simulink model "fixed_point_filter_CustArch_v9"  (R2020a)
settings: Solver=FixedStepAuto  StartTime=0  StopTime=60.5525  RelTol=1e-3
model workspace (MAT data in the model file):
  a = 0
undefined symbols (not defined in the file): fs
libraries: dsparch4 x2
settings Model: MinMaxOverflowLogging=MinMaxAndOverflow  FPTRunName=EmbeddedRun  FPTShortcutValueString='{{},{''BaselineRun_3'',1,1,1,''BaselineRun_3'','''',{},''M'',''D'',''''},{''EmbeddedRun'',1,1,1,''EmbeddedRun'','''',{},''M'','''',''''},{''BaselineRun'',1,1,1,''BaselineRun'','''',{},''M'',''D'',''''},{''BaselineRun_2'',1,1,1,''BaselineRun_2'','''',{},''M'',''D'',''''},{''EmbeddedRun_2'',1,1,1,''EmbeddedRun_2'','''',{},''M'','''',''''},{''BaselineRun_4'',1,1,1,''BaselineRun_4'','''',{},''M'',''D'',''''},{''BaselineRun_7'',1,1,1,''BaselineRun_7'','''',{},''M'',''D'',''''}}'  SimulationMode=rapid-accelerator  Creator=sbuccelli  LastModifiedBy=diflo
settings DataIOCC: SaveOutput=off  SaveTime=off
settings OptimizationCC: BlockReduction=off  ConditionallyExecuteInputs=off  DefaultParameterBehavior=Inlined
settings DebuggingCC: SignalRangeChecking=error  AlgebraicLoopMsg=error  SingleTaskRateTransMsg=error  IntegerOverflowMsg=none  ParameterDowncastMsg=none  ParameterOverflowMsg=none  ParameterPrecisionLossMsg=none  IntegerSaturationMsg=none
settings HardwareCC: ProdBitPerPointer=32  ProdBitPerSizeT=32  ProdBitPerPtrDiffT=32  ProdLargestAtomicFloat=None  ProdIntDivRoundTo=Undefined  ProdEndianess=Unspecified  ProdWordSize=32  ProdHWDeviceType=ASIC/FPGA->ASIC/FPGA  TargetBitPerPointer=64  TargetBitPerSizeT=64  TargetBitPerPtrDiffT=64  TargetLongLongMode=on  TargetIntDivRoundTo=Zero  TargetEndianess=LittleEndian  TargetWordSize=64  TargetHWDeviceType=Custom Processor->MATLAB Host Computer  ProdEqTarget=off

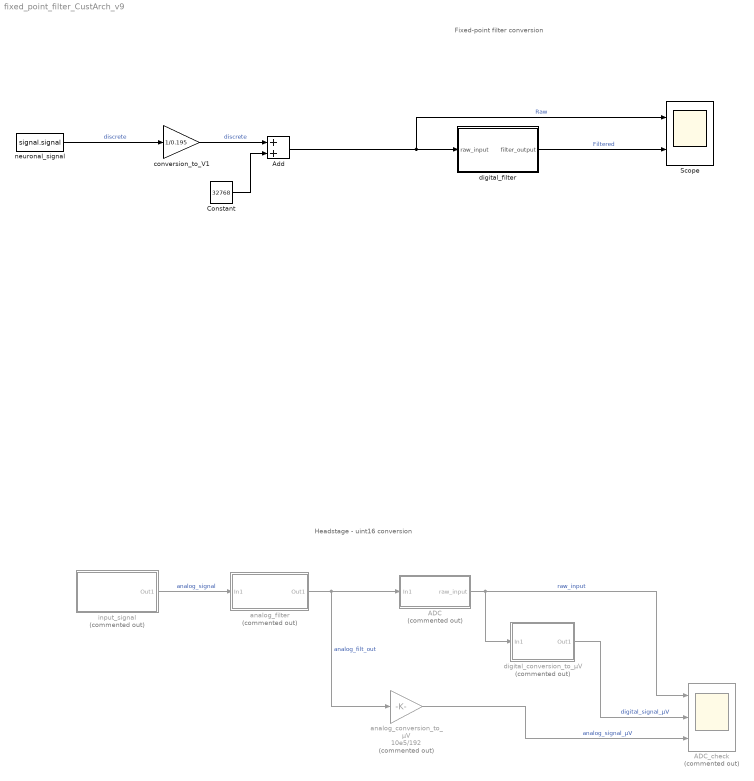
== system fixed_point_filter_CustArch_v9 ==
  note: Fixed-point filter conversion
  note: Headstage - uint16 conversion
  ADC : Subsystem  Commented=on
  ADC_check : Scope  Commented=on  NumInputPorts=3
  Add : Sum  OutDataTypeStr=uint16
  Constant : Constant  Value=32768  OutDataTypeStr=uint16  SampleTime=-1
  Scope : Scope  NumInputPorts=2
  "analog_conversion_to_µV " : Gain  Commented=on  Gain=10e5/192  SaturateOnIntegerOverflow=on  OutDataTypeStr=Inherit: Same as input  ParamDataTypeStr=Inherit: Same as input
  analog_filter : Subsystem  Commented=on
  conversion_to_V1 : Gain  Gain=1/0.195
  digital_conversion_to_µV : Subsystem  Commented=on
  digital_filter : Subsystem
  input_signal : Subsystem  Commented=on
  "neuronal_signal " : FromWorkspace  VariableName=signal.signal  SampleTime=1/fs  Interpolate=off  OutputAfterFinalValue=Setting to zero
  wires:
  input_signal/1(Out1) -> analog_filter/1(In1)  "analog_signal"
  digital_conversion_to_µV/1(Out1) -> ADC_check/2  "digital_signal_µV"
  analog_filter/1(Out1) -> "analog_conversion_to_µV "/1, ADC/1(In1)  "analog_filt_out"
  "analog_conversion_to_µV "/1 -> ADC_check/3  "analog_signal_µV"
  ADC/1(raw_input) -> ADC_check/1, digital_conversion_to_µV/1(In1)  "raw_input"
  "neuronal_signal "/1 -> conversion_to_V1/1  "discrete"
  conversion_to_V1/1 -> Add/1  "discrete"
  Constant/1 -> Add/2
  Add/1 -> digital_filter/1(raw_input), Scope/1  "Raw"
  digital_filter/1(filter_output) -> Scope/2  "Filtered"

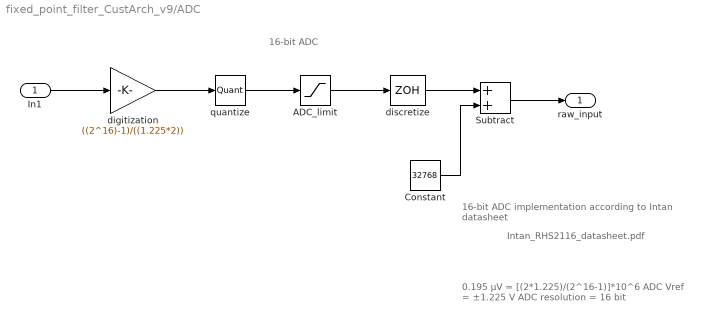
== system fixed_point_filter_CustArch_v9/ADC ==
  note: 16-bit ADC
  note: 16-bit ADC implementation according to
      | Intan datasheet
  note: 0.195 µV = [(2*1.225)/(2^16-1)]*10^6
      | ADC Vref = ±1.225 V
      | ADC resolution = 16 bit
  note: Intan_RHS2116_datasheet.pdf
  In1 : Inport
  ADC_limit : Saturate  UpperLimit=32767  LowerLimit=-32768
  Constant : Constant  Value=32768  OutDataTypeStr=double
  Subtract : Sum  OutDataTypeStr=uint16
  digitization : Gain  Gain=((2^16)-1)/((1.225*2))  SaturateOnIntegerOverflow=on  OutDataTypeStr=Inherit: Same as input  ParamDataTypeStr=Inherit: Same as input
  discretize : ZeroOrderHold  SampleTime=-1
  quantize : Quantizer  QuantizationInterval=0.000000195
  raw_input : Outport
  wires:
  quantize/1 -> ADC_limit/1
  ADC_limit/1 -> discretize/1
  In1/1 -> digitization/1
  digitization/1 -> quantize/1
  Subtract/1 -> raw_input/1
  Constant/1 -> Subtract/2
  discretize/1 -> Subtract/1

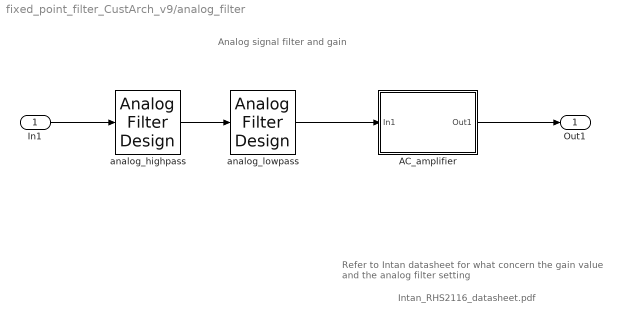
== system fixed_point_filter_CustArch_v9/analog_filter ==
  note: Intan_RHS2116_datasheet.pdf
  note: Analog signal filter and gain
  note: Refer to Intan datasheet for what concern the
      | gain value and the analog filter setting
  In1 : Inport
  AC_amplifier : Subsystem
  analog_highpass : dsparch4/Analog Filter Design  method=Butterworth  filttype=Highpass  N=1  Wlo=1/0.16  Whi=80  Rp=2  Rs=40
  analog_lowpass : dsparch4/Analog Filter Design  method=Butterworth  filttype=Lowpass  N=3  Wlo=5000/0.16  Whi=80  Rp=2  Rs=40
  Out1 : Outport
  wires:
  In1/1 -> analog_highpass/1
  AC_amplifier/1(Out1) -> Out1/1
  analog_highpass/1 -> analog_lowpass/1
  analog_lowpass/1 -> AC_amplifier/1(In1)

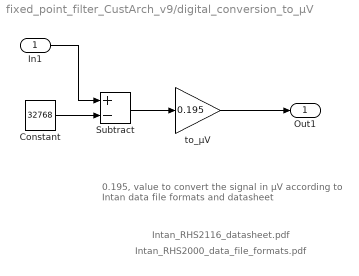
== system fixed_point_filter_CustArch_v9/digital_conversion_to_µV ==
  note: 0.195, value to convert the signal in µV
      | according to Intan data file formats and
      | datasheet
  note: Intan_RHS2116_datasheet.pdf
  note: Intan_RHS2000_data_file_formats.pdf
  In1 : Inport
  Constant : Constant  Value=32768
  Subtract : Sum  Inputs=+-
  to_µV : Gain  Gain=0.195  SaturateOnIntegerOverflow=on  OutDataTypeStr=Inherit: Same as input  ParamDataTypeStr=Inherit: Same as input
  Out1 : Outport
  wires:
  Subtract/1 -> to_µV/1
  Constant/1 -> Subtract/2
  to_µV/1 -> Out1/1
  In1/1 -> Subtract/1

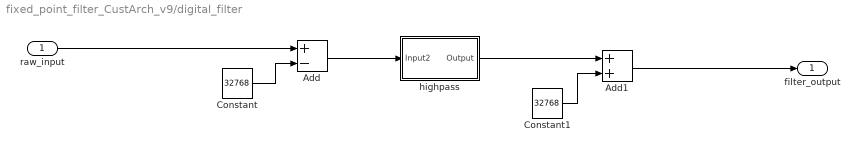
== system fixed_point_filter_CustArch_v9/digital_filter ==
  raw_input : Inport  OutDataTypeStr=uint16  LockScale=on
  Add : Sum  Inputs=+-  OutDataTypeStr=fixdt(1,16,-3)  SaturateOnIntegerOverflow=on  LockScale=on
  Add1 : Sum  OutDataTypeStr=uint16  SaturateOnIntegerOverflow=on  LockScale=on
  Constant : Constant  Value=32768  OutDataTypeStr=fixdt(0,16,0)  SampleTime=-1
  Constant1 : Constant  Value=32768  OutDataTypeStr=fixdt(0,16,0)  SampleTime=-1
  highpass : Subsystem  Tag=BlockMethodSubSystem
  filter_output : Outport  LockScale=on
  wires:
  Constant/1 -> Add/2
  Add/1 -> highpass/1(Input2)
  Constant1/1 -> Add1/2
  highpass/1(Output) -> Add1/1
  raw_input/1 -> Add/1
  Add1/1 -> filter_output/1

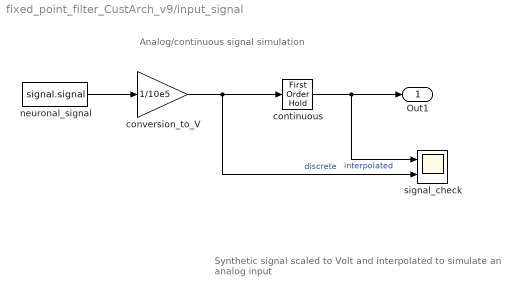
== system fixed_point_filter_CustArch_v9/input_signal ==
  note: Synthetic signal scaled to Volt and interpolated to
      | simulate an analog input
  note: Analog/continuous signal simulation
  continuous : FirstOrderHold  ErrorTolerance=inf
  conversion_to_V : Gain  Gain=1/10e5
  "neuronal_signal " : FromWorkspace  VariableName=signal.signal  SampleTime=1/fs
  signal_check : Scope  NumInputPorts=2
  Out1 : Outport
  wires:
  "neuronal_signal "/1 -> conversion_to_V/1
  conversion_to_V/1 -> continuous/1, signal_check/2  "discrete"
  continuous/1 -> signal_check/1, Out1/1  "interpolated"

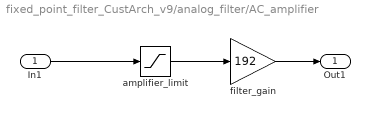
== system fixed_point_filter_CustArch_v9/analog_filter/AC_amplifier ==
  In1 : Inport
  amplifier_limit : Saturate  UpperLimit=5e-3  LowerLimit=-5e-3
  filter_gain : Gain  Gain=192  SaturateOnIntegerOverflow=on  OutDataTypeStr=Inherit: Same as input  ParamDataTypeStr=Inherit: Same as input
  Out1 : Outport
  wires:
  filter_gain/1 -> Out1/1
  In1/1 -> amplifier_limit/1
  amplifier_limit/1 -> filter_gain/1

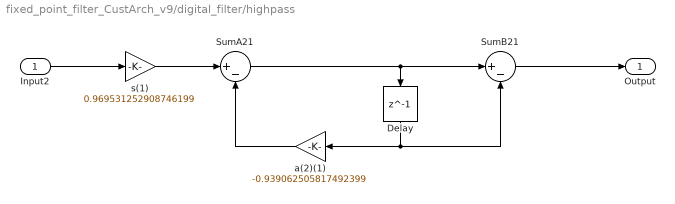
== system fixed_point_filter_CustArch_v9/digital_filter/highpass ==
  Input2 : Inport  OutDataTypeStr=fixdt(1,16,-3)
  Delay : Delay  DelayLength=1  InitialCondition=0
  SumA21 : Sum  Inputs=|+-  OutDataTypeStr=fixdt(1,16,-3)  RndMeth=Nearest  SaturateOnIntegerOverflow=on
  SumB21 : Sum  Inputs=|+-  OutDataTypeStr=fixdt(1,16,-3)  RndMeth=Nearest  SaturateOnIntegerOverflow=on
  a(2)(1) : Gain  Gain=-0.939062505817492399  ParamDataTypeStr=fixdt(1,32,31)  OutDataTypeStr=fixdt(1,16,-3)  RndMeth=Nearest  SaturateOnIntegerOverflow=on
  s(1) : Gain  Gain=0.969531252908746199  ParamDataTypeStr=fixdt(0,32,32)  OutDataTypeStr=fixdt(1,16,-3)  RndMeth=Nearest  SaturateOnIntegerOverflow=on
  Output : Outport
  wires:
  SumB21/1 -> Output/1
  SumA21/1 -> SumB21/1, Delay/1
  s(1)/1 -> SumA21/1
  Input2/1 -> s(1)/1
  a(2)(1)/1 -> SumA21/2
  Delay/1 -> SumB21/2, a(2)(1)/1
